simulink model "Prob_1"  (R2020b)
settings: Solver=VariableStepAuto  StartTime=0.0  StopTime=10.0  RelTol=1e-3
undefined symbols (not defined in the file): b, K1, K12, M1, M2
settings Model: Creator=Lenovo  LastModifiedBy=Lenovo

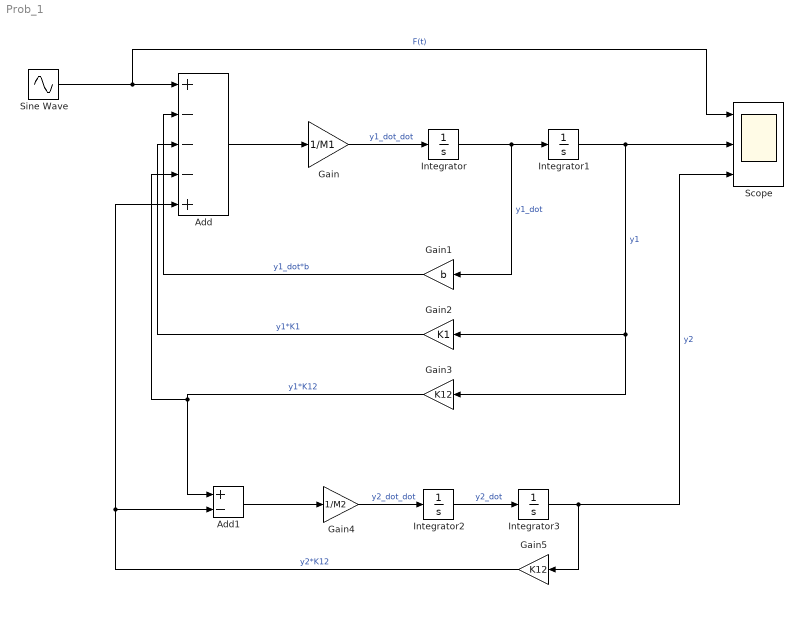
== system Prob_1 ==
  Add : Sum  Inputs=+---+
  Add1 : Sum  Inputs=+-
  Gain : Gain  Gain=1/M1
  Gain1 : Gain  Gain=b
  Gain2 : Gain  Gain=K1
  Gain3 : Gain  Gain=K12
  Gain4 : Gain  Gain=1/M2
  Gain5 : Gain  Gain=K12
  Integrator{,1..3} (4 alike) : Integrator
  Scope : Scope  NumInputPorts=3
  Sine Wave : Sin  Amplitude=2  Frequency=10  SampleTime=0
  wires:
  Gain5/1 -> Add/5, Add1/2  "y2*K12"
  Gain4/1 -> Integrator2/1  "y2_dot_dot"
  Integrator2/1 -> Integrator3/1  "y2_dot"
  Integrator3/1 -> Scope/3, Gain5/1  "y2"
  Gain3/1 -> Add1/1, Add/4  "y1*K12"
  Add1/1 -> Gain4/1
  Gain1/1 -> Add/2  "y1_dot*b"
  Integrator/1 -> Gain1/1, Integrator1/1  "y1_dot"
  Gain/1 -> Integrator/1  "y1_dot_dot"
  Integrator1/1 -> Scope/2, Gain2/1, Gain3/1  "y1"
  Add/1 -> Gain/1
  Gain2/1 -> Add/3  "y1*K1"
  Sine Wave/1 -> Scope/1, Add/1  "F(t)"
